simulink model "beta_estimator_velocity"  (R2022a)
settings: Solver=VariableStepAuto  StartTime=0.0  StopTime=10  FixedStep=1e-3  RelTol=1e-6  AbsTol=1e-10
values from neighbouring files (symbols this model uses):
  Kp = 100    [test_beta_estimator_compare.m]    (also in test_beta_estimator_velocity.m)
  Ts = 0.001    [test_beta_estimator_acceleration.m]    (also in test_beta_estimator_compare.m; test_beta_estimator_velocity.m)
  x0_vel = [0,0,0]    [test_beta_estimator_compare.m]    (also in test_beta_estimator_velocity.m)
undefined symbols (not defined in the file or in its folder): DiscIntNeverNeededParam
settings Model: Creator=bascetta  LastModifiedBy=bascetta
settings SolverCC: AlgebraicLoopSolver=TrustRegion
settings DataIOCC: SaveOutput=off  SignalLogging=off  DSMLogging=off  SaveTime=off  ReturnWorkspaceOutputs=off
settings OptimizationCC: DefaultParameterBehavior=Inlined  PassReuseOutputArgsAs=Individual arguments  MaxStackSize=64  EfficientTunableParamExpr=on
settings DebuggingCC: ParameterTunabilityLossMsg=error  UnconnectedInputMsg=warning  UnconnectedOutputMsg=warning  UnconnectedLineMsg=warning  SFMachineParentedDataDiag=warning  ArithmeticOperatorsInVariantConditions=warning
settings HardwareCC: ProdBitPerPointer=32  ProdBitPerSizeT=32  ProdBitPerPtrDiffT=32  ProdLargestAtomicFloat=None  ProdIntDivRoundTo=Undefined  ProdEndianess=Unspecified  ProdWordSize=32  ProdHWDeviceType=Generic->Unspecified (assume 32-bit Generic)
settings SFSimCC: SimUseLocalCustomCode=off  MATLABDynamicMemAlloc=off  CustomCodeUndefinedFunction=UseInterfaceOnly
settings RTWCC: SystemTargetFile=ert.tlc  TemplateMakefile=ert_default_tmf  GenerateReport=on  RTWUseLocalCustomCode=off  Toolchain=Catkin  IncludeHyperlinkInReport=on  LaunchReport=on  GenerateTraceInfo=on  GenerateTraceReport=on  GenerateTraceReportSl=on  GenerateTraceReportSf=on  GenerateTraceReportEml=on  DLArmComputeVersion=19.05
settings CodeAppCC: ForceParamTrailComments=on  IgnoreCustomStorageClasses=off  OperatorAnnotations=on  SimulinkDataObjDesc=on  SFDataObjDesc=on  MATLABFcnDesc=on  InsertBlockDesc=on  StateflowObjectComments=on  MATLABSourceComments=on
settings ERTTargetCC: ERTCustomFileTemplate=example_file_process.tlc

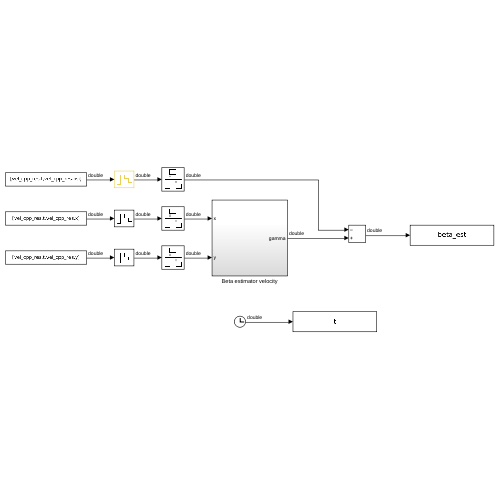
[thumbnail: Simulink's stored preview of the top-level diagram]
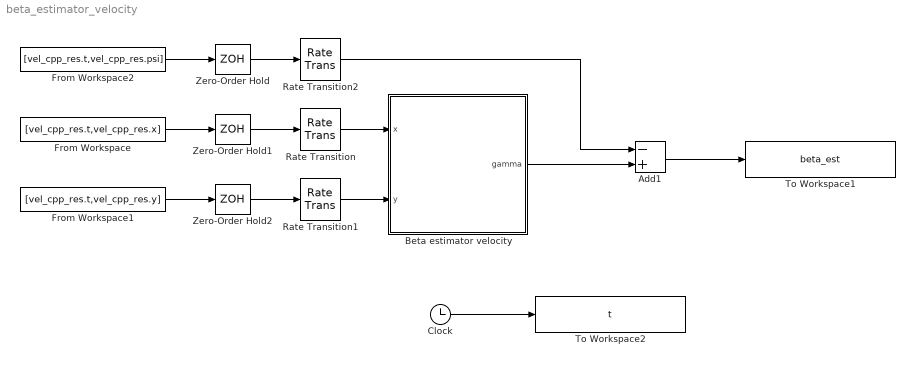
== system beta_estimator_velocity ==
  Add1 : Sum  Inputs=-+
  Beta estimator velocity : Subsystem
  Clock : Clock
  From Workspace : FromWorkspace  VariableName=[vel_cpp_res.t,vel_cpp_res.x]  OutputAfterFinalValue=Holding final value
  From Workspace1 : FromWorkspace  VariableName=[vel_cpp_res.t,vel_cpp_res.y]  OutputAfterFinalValue=Holding final value
  From Workspace2 : FromWorkspace  VariableName=[vel_cpp_res.t,vel_cpp_res.psi]  OutputAfterFinalValue=Holding final value
  Rate Transition : RateTransition  OutPortSampleTime=Ts
  Rate Transition1 : RateTransition  OutPortSampleTime=Ts
  Rate Transition2 : RateTransition  OutPortSampleTime=Ts
  To Workspace1 : ToWorkspace  VariableName=beta_est  SampleTime=Ts
      settings: Save2DSignal=2-D array (concatenate along first dimension)
  To Workspace2 : ToWorkspace  VariableName=t  SampleTime=0.001
      settings: Save2DSignal=2-D array (concatenate along first dimension)
  Zero-Order Hold : ZeroOrderHold  SampleTime=0.01
  Zero-Order Hold1 : ZeroOrderHold  SampleTime=0.01
  Zero-Order Hold2 : ZeroOrderHold  SampleTime=0.01
  wires:
  Beta estimator velocity/1(gamma) -> Add1/2
  Add1/1 -> To Workspace1/1
  From Workspace1/1 -> Zero-Order Hold2/1
  From Workspace2/1 -> Zero-Order Hold/1
  From Workspace/1 -> Zero-Order Hold1/1
  Clock/1 -> To Workspace2/1
  Rate Transition1/1 -> Beta estimator velocity/2(y)
  Rate Transition/1 -> Beta estimator velocity/1(x)
  Rate Transition2/1 -> Add1/1
  Zero-Order Hold/1 -> Rate Transition2/1
  Zero-Order Hold2/1 -> Rate Transition1/1
  Zero-Order Hold1/1 -> Rate Transition/1

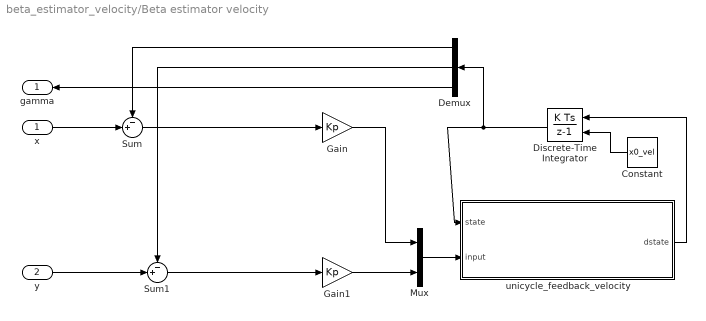
== system beta_estimator_velocity/Beta estimator velocity ==
  x : Inport
  y : Inport  Port=2
  Constant : Constant  Value=x0_vel
  Demux : Demux  Outputs=3
  Discrete-Time Integrator : DiscreteIntegrator  InitialConditionSource=external  SampleTime=Ts  ICPrevOutput=DiscIntNeverNeededParam  ICPrevScaledInput=DiscIntNeverNeededParam
  Gain : Gain  Gain=Kp
  Gain1 : Gain  Gain=Kp
  Mux : Mux  Inputs=2
  Sum : Sum  Inputs=-+|
  Sum1 : Sum  Inputs=-+|
  unicycle_feedback_velocity : MATLAB Function  TreatAsAtomicUnit=on
  gamma : Outport  VectorParamsAs1DForOutWhenUnconnected=off
  wires:
  Demux/3 -> gamma/1
  y/1 -> Sum1/2
  Demux/1 -> Sum/1
  Gain1/1 -> Mux/2
  Gain/1 -> Mux/1
  Mux/1 -> unicycle_feedback_velocity/2(input)
  Demux/2 -> Sum1/1
  x/1 -> Sum/2
  unicycle_feedback_velocity/1(dstate) -> Discrete-Time Integrator/1
  Discrete-Time Integrator/1 -> Demux/1, unicycle_feedback_velocity/1(state)
  Sum1/1 -> Gain1/1
  Sum/1 -> Gain/1
  Constant/1 -> Discrete-Time Integrator/2

== matlab function beta_estimator_velocity/Beta estimator velocity/unicycle_feedback_velocity ==
  data: state input size=3; dstate output size=3; input input size=2; p parameter size=1
function dstate = unicycle_feedback_velocity(state,input,p)

% State and input variables
x     = state(1);
y     = state(2);
gamma = state(3); % theta+beta

vxp   = input(1);
vyp   = input(2);


% Model equations
dstate = zeros(3,1);
dstate(1) = vxp*cos(gamma)^2+vyp*sin(gamma)*cos(gamma);
dstate(2) = vxp*sin(gamma)*cos(gamma)+vyp*sin(gamma)^2;
dstate(3) = (vyp*cos(gamma)-vxp*sin(gamma))/p;
